simulink model "controller"  (R2019b)
settings: Solver=FixedStepAuto  StartTime=0.0  StopTime=t_end  FixedStep=0.01  MaxStep=.1  RelTol=1e-3
values from neighbouring files (symbols this model uses):
  K = zeros(1,2)    [duffing_init.m]    (also in duffing_trim.m)
  Ts = 10*dt    (= 0.1)    [duffing_init.m]    (also in duffing_trim.m = 0.3)
settings Model: Creator=enrique.babio  LastModifiedBy=enrique.babio
settings DataIOCC: SaveOutput=off  SaveState=on  SaveTime=off

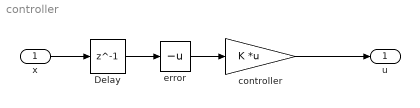
== system controller ==
  x : Inport  OutDataTypeStr=double  PortDimensions=2  SampleTime=0
  Delay : Delay  DelayLength=1  SampleTime=Ts
  controller : Gain  Gain=K  Multiplication=Matrix(K*u)
  error : UnaryMinus
  u : Outport  OutDataTypeStr=double  PortDimensions=1  SampleTime=[0.29999999999999999,0]
  wires:
  error/1 -> controller/1
  controller/1 -> u/1
  x/1 -> Delay/1
  Delay/1 -> error/1
